simulink model "plant_model"  (Simulink 7.5)
settings: Solver=ode45  StartTime=0.0  StopTime=20  RelTol=1e-3
values from neighbouring files (symbols this model uses):
  d1bar = 0    [script.m]
  d2bar = 0    [script.m]
  Ibar = sign(wbar)*Ifr + b*abs(wbar)*wbar/K + d1bar    [script.m]
  Ubar = R*Ibar+K*wbar-d2bar    [script.m]
  wbar = 300    [script.m]
undefined symbols (not defined in the file or in its folder): syss
libraries: cstblocks x1, simulink x1
settings Model: Creator=PhM  LastModifiedBy=PhM
settings OptimizationCC: InitFltsAndDblsToZero=on
settings DebuggingCC: SaveWithParameterizedLinksMsg=none  SignalResolutionControl=TryResolveAllWithWarning  MultiTaskDSMMsg=warning  MultiTaskCondExecSysMsg=none  StrictBusMsg=None
settings RTWCC: IncludeERTFirstTime=on
settings GRTTargetCC: TargetFcnLib=ansi_tfl_tmw.mat

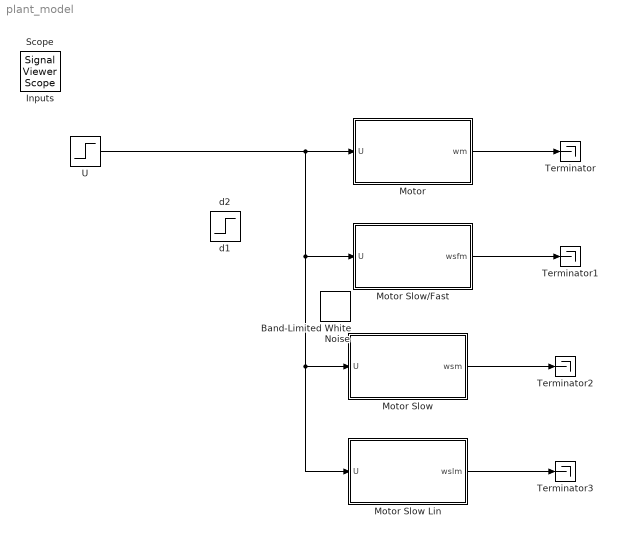
== system plant_model ==
  Motor : Subsystem
  Motor Slow : Subsystem
  Motor Slow Lin : Subsystem
  Motor Slow/Fast : Subsystem
  Terminator{,1..3} (4 alike) : Terminator
  U : Step  Time=5  Before=Ubar  After=Ubar+1  SampleTime=0
  Band-Limited White Noise : simulink/Sources/Band-Limited White Noise  IOType=siggen  SystemSampleTime=-1  Cov=[0.1]  Ts=1e-2  seed=[23341]
  Inputs : SignalViewerScope  IOType=viewer  NumInputPorts=3  LegendLocations=|  RefreshTime=0.035000
      | 240.3333           653            66      20.33333
      | 236.8333         431.5            70      20.33333
      | 236.8333         211.5            70      20.33333
      settings: ShowLegends=on  TimeRange=20  YMin=4.5~0~0  YMax=6.000000000000001~1~1
  Scope : SignalViewerScope  IOType=viewer  NumInputPorts=3  RefreshTime=0.035000
      settings: TimeRange=20  YMin=280~300~2  YMax=400~380~5.5
  d1 : Step  IOType=siggen  Time=10  Before=d1bar  After=d1bar+1  SampleTime=0
  d2 : Step  IOType=siggen  Time=15  Before=d2bar  After=d2bar+1  SampleTime=0
  wires:
  Motor/1(wm) -> Terminator/1
  U/1 -> Motor/1(U), Motor Slow/Fast/1(U), Motor Slow/1(U), Motor Slow Lin/1(U)
  Motor Slow/1(wsm) -> Terminator2/1
  Motor Slow Lin/1(wslm) -> Terminator3/1
  Motor Slow/Fast/1(wsfm) -> Terminator1/1

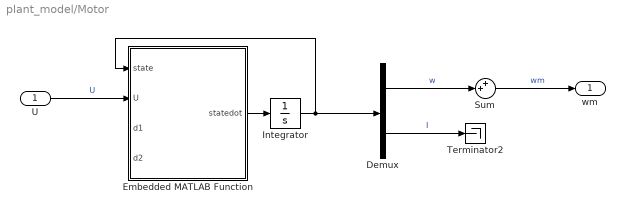
== system plant_model/Motor ==
  U : Inport  OutDataType=sfix(16)  OutScaling=2^0
  Demux : Demux  Outputs=2
  Embedded MATLAB Function : Stateflow chart  TreatAsAtomicUnit=on
  Integrator : Integrator  InitialCondition=[wbar; Ibar]
  Sum : Sum  Inputs=++|  OutDataType=sfix(16)  OutScaling=2^0
  Terminator2 : Terminator
  wm : Outport  OutDataType=sfix(16)  OutScaling=2^0
  wires:
  Embedded MATLAB Function/1(statedot) -> Integrator/1
  Integrator/1 -> Embedded MATLAB Function/1(state), Demux/1
  U/1 -> Embedded MATLAB Function/2(U)  "U"
  Demux/1 -> Sum/2  "w"
  Demux/2 -> Terminator2/1  "I"
  Sum/1 -> wm/1  "wm"

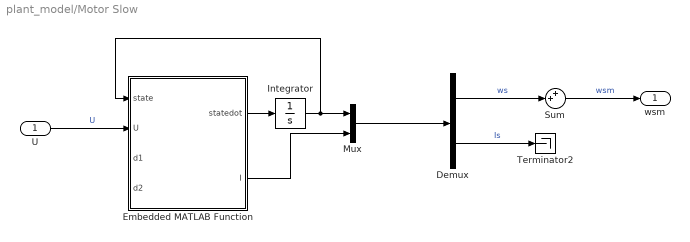
== system plant_model/Motor Slow ==
  U : Inport  OutDataType=sfix(16)  OutScaling=2^0
  Demux : Demux  Outputs=2
  Embedded MATLAB Function : Stateflow chart  TreatAsAtomicUnit=on
  Integrator : Integrator  InitialCondition=[wbar]
  Mux : Mux  Inputs=2
  Sum : Sum  Inputs=++|  OutDataType=sfix(16)  OutScaling=2^0
  Terminator2 : Terminator
  wsm : Outport  OutDataType=sfix(16)  OutScaling=2^0
  wires:
  Embedded MATLAB Function/1(statedot) -> Integrator/1
  Integrator/1 -> Embedded MATLAB Function/1(state), Mux/1
  U/1 -> Embedded MATLAB Function/2(U)  "U"
  Embedded MATLAB Function/2(I) -> Mux/2
  Demux/1 -> Sum/2  "ws"
  Demux/2 -> Terminator2/1  "Is"
  Sum/1 -> wsm/1  "wsm"
  Mux/1 -> Demux/1

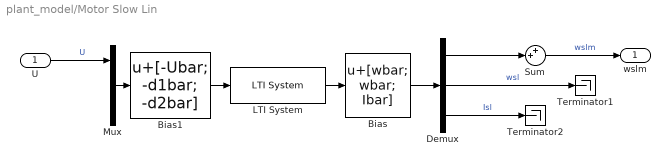
== system plant_model/Motor Slow Lin ==
  U : Inport  OutDataType=sfix(16)  OutScaling=2^0
  Bias : Bias  Bias=[wbar; wbar; Ibar]
  Bias1 : Bias  Bias=[-Ubar; -d1bar; -d2bar]
  Demux : Demux  Outputs=3
  LTI System : cstblocks/LTI System  SystemSampleTime=-1  sys=syss(:,:,2)  IC=0
  Mux : Mux  Inputs=3
  Sum : Sum  Inputs=++|  OutDataType=sfix(16)  OutScaling=2^0
  Terminator1 : Terminator
  Terminator2 : Terminator
  wslm : Outport  OutDataType=sfix(16)  OutScaling=2^0
  wires:
  Sum/1 -> wslm/1  "wslm"
  Demux/3 -> Terminator2/1  "Isl"
  Demux/2 -> Terminator1/1  "wsl"
  Demux/1 -> Sum/2
  U/1 -> Mux/1  "U"
  Mux/1 -> Bias1/1
  LTI System/1 -> Bias/1
  Bias/1 -> Demux/1
  Bias1/1 -> LTI System/1

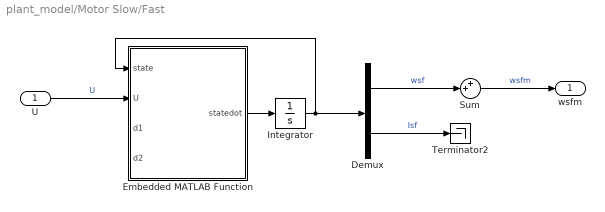
== system plant_model/Motor Slow/Fast ==
  U : Inport  OutDataType=sfix(16)  OutScaling=2^0
  Demux : Demux  Outputs=2
  Embedded MATLAB Function : Stateflow chart  TreatAsAtomicUnit=on
  Integrator : Integrator  InitialCondition=[wbar; Ibar]
  Sum : Sum  Inputs=++|  OutDataType=sfix(16)  OutScaling=2^0
  Terminator2 : Terminator
  wsfm : Outport  OutDataType=sfix(16)  OutScaling=2^0
  wires:
  Embedded MATLAB Function/1(statedot) -> Integrator/1
  Integrator/1 -> Embedded MATLAB Function/1(state), Demux/1
  U/1 -> Embedded MATLAB Function/2(U)  "U"
  Demux/1 -> Sum/2  "wsf"
  Demux/2 -> Terminator2/1  "Isf"
  Sum/1 -> wsfm/1  "wsfm"

== matlab function Motor Slow/Fast/Embedded MATLAB Function ==
  data: state input double; statedot output double; U input double; d1 input double; d2 input double
function statedot = fcn(state,U,d1,d2)
% This block supports an embeddable subset of the MATLAB language.
% See the help menu for details. 

R = 0.56;
L = 0.4e-3*10;
Ifr = 0.4;
K = 1.19e-2;
J = 3.45e-5;
b = 2.4e-7;

w = state(1);
I = state(2);

wdot = (K/R*U  - sign(w)*K*Ifr - (K^2/R+abs(w)*b)*w + K*(d2/R-d1) )/J;
Idot = (-R*I-K*w+U+d2)/L;

statedot = [wdot; Idot];

== matlab function Motor/Embedded MATLAB Function ==
  data: state input double; statedot output double; U input double; d1 input double; d2 input double
function statedot = fcn(state,U,d1,d2)
% This block supports an embeddable subset of the MATLAB language.
% See the help menu for details. 

R = 0.56;
L = 0.4e-3*10;
Ifr = 0.4;
K = 1.19e-2;
J = 3.45e-5;
b = 2.4e-7;

w = state(1);
I = state(2);

wdot = (K*I  - sign(w)*K*Ifr - b*abs(w)*w - K*d1)/J;
Idot = (-R*I-K*w+U+d2)/L;

statedot = [wdot; Idot];

== matlab function Motor Slow/Embedded MATLAB Function ==
  data: state input double; statedot output double; U input double; d1 input double; d2 input double; I output double
function [statedot,I] = fcn(state,U,d1,d2)
% This block supports an embeddable subset of the MATLAB language.
% See the help menu for details. 

R = 0.56;
L = 0.4e-3*10;
Ifr = 0.4;
K = 1.19e-2;
J = 3.45e-5;
b = 2.4e-7;

w = state(1);

wdot = (K/R*U  - sign(w)*K*Ifr - (K^2/R+abs(w)*b)*w + K*(d2/R-d1) )/J;

statedot = [wdot];
I = (U-K*w+d2)/R;
